simulink model "reference_sl"  (R2014b)
settings: Solver=ode45  StartTime=0.0  StopTime=20  RelTol=1e-3
values from neighbouring files (symbols this model uses):
  b = 0.00007892    (= 7.892e-05)    [origin.m]    (also in reference.m)
  c = 0.063    [origin.m]    (also in reference.m = 0.63)
  g = 9.8    [origin.m]    (also in reference.m = 9.81)
  I = 0.0007176    [reference.m]
  l = 0.2    [origin.m]    (also in reference.m)
  M = 0.136    [origin.m]    (also in reference.m)
  m = 0.1    [origin.m]    (also in reference.m)
libraries: simulink x1
settings Model: Creator=Admin  LastModifiedBy=Admin

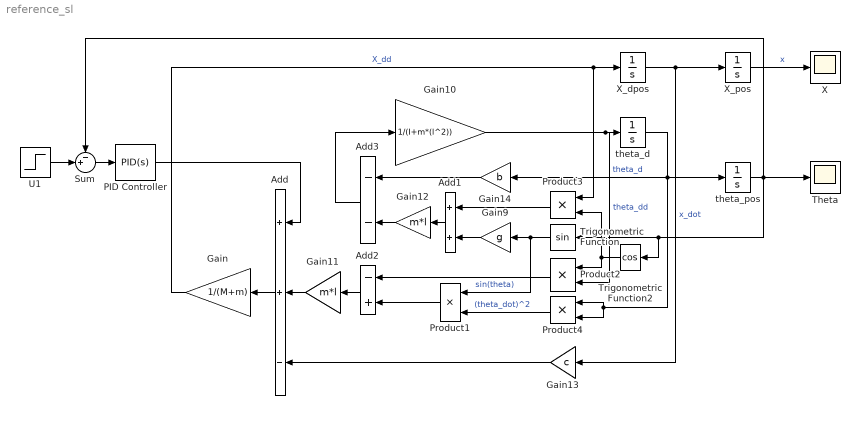
== system reference_sl ==
  Add : Sum  Inputs=++-
  Add1 : Sum
  Add2 : Sum  Inputs=-+
  Add3 : Sum  Inputs=--
  Gain : Gain  Gain=1/(M+m)
  Gain10 : Gain  Gain=1/(I+m*(l^2))
  Gain11 : Gain  Gain=m*l
  Gain12 : Gain  Gain=m*l
  Gain13 : Gain  Gain=c
  Gain14 : Gain  Gain=b
  Gain9 : Gain  Gain=g
  PID Controller : simulink/Continuous/PID Controller  Controller=PID  TimeDomain=Continuous-time  SampleTime=-1  IntegratorMethod=Forward Euler  FilterMethod=Forward Euler  Form=Parallel  P=0.1  I=1  D=0  N=0  InitialConditionSource=internal  InitialConditionForIntegrator=0  InitialConditionForFilter=0  ExternalReset=none  LimitOutput=off  UpperSaturationLimit=inf  LowerSaturationLimit=-inf  LinearizeAsGain=on  AntiWindupMode=none  Kb=1  TrackingMode=off  Kt=1  PParamMin=[]  PParamMax=[]  IParamMin=[]  IParamMax=[]  DParamMin=[]  DParamMax=[]  NParamMin=[]  NParamMax=[]  KbParamMin=[]  KbParamMax=[]  KtParamMin=[]  KtParamMax=[]  POutMin=[]  POutMax=[]  IOutMin=[]  IOutMax=[]  DOutMin=[]  DOutMax=[]  NOutMin=[]  NOutMax=[]  KbOutMin=[]  KbOutMax=[]  KtOutMin=[]  KtOutMax=[]  IntegratorOutMin=[]  IntegratorOutMax=[]  FilterOutMin=[]  FilterOutMax=[]  SumOutMin=[]  SumOutMax=[]  SumI1OutMin=[]  SumI1OutMax=[]  SumI2OutMin=[]  SumI2OutMax=[]  SumI3OutMin=[]  SumI3OutMax=[]  SumDOutMin=[]  SumDOutMax=[]  SaturationOutMin=[]  SaturationOutMax=[]  IntegratorContinuousStateAttributes=''  IntegratorStateMustResolveToSignalObject=off  IntegratorRTWStateStorageClass=Auto  FilterContinuousStateAttributes=''  FilterStateMustResolveToSignalObject=off  FilterRTWStateStorageClass=Auto  DifferentiatorICPrevScaledInput=0  DifferentiatorOutMin=[]  DifferentiatorOutMax=[]  UseFilter=on
  Product{1..4} (4 alike) : Product
  Sum : Sum  Inputs=-+|
  Theta : Scope
      settings: TimeRange=1.17741935483871  YMin=2.541237113402061  YMax=2.932989690721648
  Trigonometric Function : Trigonometry
  Trigonometric Function2 : Trigonometry  Operator=cos
  U1 : Step  Time=0.1  After=3.14  SampleTime=0
  X : Scope
      settings: TimeRange=10  YMin=-4  YMax=1
  X_dpos : Integrator
  X_pos : Integrator  InitialCondition=0.2
  theta_d : Integrator
  theta_pos : Integrator  InitialCondition=160*(pi/180)
  wires:
  Gain13/1 -> Add/3
  Add2/1 -> Gain11/1
  Add3/1 -> Gain10/1
  Trigonometric Function2/1 -> Product3/2, Product2/1
  Trigonometric Function/1 -> Product1/1, Gain9/1  "sin(theta)"
  Gain11/1 -> Add/2
  theta_d/1 -> Product4/2, Product4/1, Gain14/1, theta_pos/1  "theta_d"
  Product3/1 -> Add1/1
  Product1/1 -> Add2/2
  Gain12/1 -> Add3/2
  Product4/1 -> Product1/2  "(theta_dot)^2"
  X_pos/1 -> X/1  "x"
  Product2/1 -> Add2/1
  Gain/1 -> X_dpos/1, Product3/1  "X_dd"
  Add/1 -> Gain/1
  Gain10/1 -> Product2/2, theta_d/1  "theta_dd"
  Gain14/1 -> Add3/1
  Gain9/1 -> Add1/2
  X_dpos/1 -> X_pos/1, Gain13/1  "x_dot"
  Add1/1 -> Gain12/1
  theta_pos/1 -> Sum/1, Theta/1, Trigonometric Function2/1, Trigonometric Function/1
  U1/1 -> Sum/2
  Sum/1 -> PID Controller/1
  PID Controller/1 -> Add/1
